simulink model "pid_linear"  (R2018a)
settings: Solver=ode4  StartTime=0.0  StopTime=4  FixedStep=0.001  RelTol=1e-3
libraries: cstblocks x20
settings Model: Creator=adios  LastModifiedBy=adios

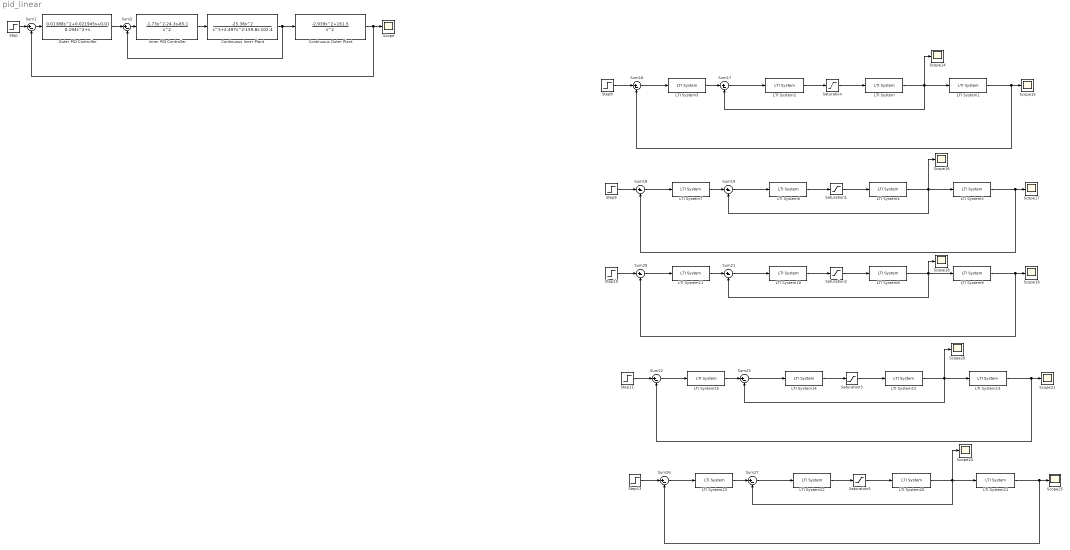
== system pid_linear ==
  Continuous Inner Plant : TransferFcn  Numerator=[-25.36 0 0]  Denominator=[1 2.497 -159.8 -102.4]
  Continuous Outer Plant : TransferFcn  Numerator=[-2.939 0 161.5]  Denominator=[1 0 0]
  Inner PID Controller : TransferFcn  Numerator=[-1.73 -24.3 -85.1]  Denominator=[1 0 0]
  LTI System : cstblocks/LTI System  sys=inn1  IC=[]
  LTI System1 : cstblocks/LTI System  sys=outer1  IC=[]
  LTI System10 : cstblocks/LTI System  sys=id3  IC=[]
  LTI System11 : cstblocks/LTI System  sys=od3  IC=[]
  LTI System12 : cstblocks/LTI System  sys=inn4  IC=[]
  LTI System13 : cstblocks/LTI System  sys=outer4  IC=[]
  LTI System14 : cstblocks/LTI System  sys=id4  IC=[]
  LTI System15 : cstblocks/LTI System  sys=od4  IC=[]
  LTI System2 : cstblocks/LTI System  sys=id1  IC=[]
  LTI System20 : cstblocks/LTI System  sys=inn5  IC=[]
  LTI System21 : cstblocks/LTI System  sys=outer5  IC=[]
  LTI System22 : cstblocks/LTI System  sys=id5  IC=[]
  LTI System23 : cstblocks/LTI System  sys=od5  IC=[]
  LTI System3 : cstblocks/LTI System  sys=od1  IC=[]
  LTI System4 : cstblocks/LTI System  sys=inn2  IC=[]
  LTI System5 : cstblocks/LTI System  sys=outer2  IC=[]
  LTI System6 : cstblocks/LTI System  sys=id2  IC=[]
  LTI System7 : cstblocks/LTI System  sys=od2  IC=[]
  LTI System8 : cstblocks/LTI System  sys=inn3  IC=[]
  LTI System9 : cstblocks/LTI System  sys=outer3  IC=[]
  Outer PID Controller : TransferFcn  Numerator=[0.01388 0.021945 0.01]  Denominator=[0.194 1 0]
  Saturation{,1..3,5} (5 alike) : Saturate  UpperLimit=30  LowerLimit=-30
  Scope{,14..21,24..25} (11 alike) : Scope
  Step : Step  Time=0  SampleTime=0
  Step{8..11,13} (5 alike) : Step  Time=0  After=0.1  SampleTime=0
  Sum{1..2,16..23,26..27} (12 alike) : Sum  Inputs=|+-
  wires:
  Inner PID Controller/1 -> Continuous Inner Plant/1
  Sum2/1 -> Inner PID Controller/1
  Continuous Inner Plant/1 -> Continuous Outer Plant/1, Sum2/2
  Step/1 -> Sum1/1
  Sum1/1 -> Outer PID Controller/1
  Outer PID Controller/1 -> Sum2/1
  Continuous Outer Plant/1 -> Sum1/2, Scope/1
  Sum17/1 -> LTI System2/1
  LTI System3/1 -> Sum17/1
  LTI System2/1 -> Saturation/1
  Step8/1 -> Sum16/1
  Sum16/1 -> LTI System3/1
  LTI System/1 -> Sum17/2, Scope14/1, LTI System1/1
  LTI System1/1 -> Scope15/1, Sum16/2
  Saturation/1 -> LTI System/1
  Step9/1 -> Sum18/1
  Sum18/1 -> LTI System7/1
  LTI System5/1 -> Scope17/1, Sum18/2
  LTI System7/1 -> Sum19/1
  LTI System4/1 -> Sum19/2, Scope16/1, LTI System5/1
  Sum19/1 -> LTI System6/1
  Saturation1/1 -> LTI System4/1
  LTI System6/1 -> Saturation1/1
  Sum21/1 -> LTI System10/1
  LTI System10/1 -> Saturation2/1
  Saturation2/1 -> LTI System8/1
  LTI System8/1 -> Sum21/2, Scope18/1, LTI System9/1
  LTI System11/1 -> Sum21/1
  Step10/1 -> Sum20/1
  LTI System9/1 -> Scope19/1, Sum20/2
  Sum20/1 -> LTI System11/1
  Sum23/1 -> LTI System14/1
  LTI System14/1 -> Saturation3/1
  Saturation3/1 -> LTI System12/1
  LTI System12/1 -> Sum23/2, Scope20/1, LTI System13/1
  LTI System15/1 -> Sum23/1
  Step11/1 -> Sum22/1
  LTI System13/1 -> Scope21/1, Sum22/2
  Sum22/1 -> LTI System15/1
  Step13/1 -> Sum26/1
  LTI System21/1 -> Scope25/1, Sum26/2
  Sum26/1 -> LTI System23/1
  Sum27/1 -> LTI System22/1
  LTI System22/1 -> Saturation5/1
  LTI System20/1 -> Sum27/2, Scope24/1, LTI System21/1
  Saturation5/1 -> LTI System20/1
  LTI System23/1 -> Sum27/1
